simulink model "gtm_aeromodel"  (Simulink 7.2)
settings: Solver=ode45  StartTime=0.0  StopTime=10.0  RelTol=1e-3
undefined symbols (not defined in the file or in its folder): A_BLCG, A_BW, A_CW, A_FSCG, A_FSREF_in, A_SW, A_WLCG, A_WLREF, ALPHA0, bclowb, bclowbx_FMACH, bcmowb, bcmowbx_FHP, bcmowby_FMACH, cda, cdax_FLPDEF, cddr, cddrx_FMACH, cdo, cdox_FLPDEF, cdt1, cdt1x_mach, cdt2, cdt2x_mach, cdto, cdtox_mach, cdwb, cdwbx_FALPHA, cdwby_FMACH, clat, clatfr, clatfrx_FHP, clatfry_FMACH, clatx_mach, clawbfr, clawbfrx_FHP, clawbfry_FMACH, cldefr, cldefrx_FHP, cldefry_FMACH, cldtab, cldtabx_FMACH, clqwb, clqwbfr, clqwbfrx_FHP, clqwbfry_FMACH, clqwbx_mach, cltdd, cltddx_FHP, cltddy_FMACH, clwb, clwbtdd, clwbtddx_FHP, clwbtddy_FMACH, clwbx_FALPHA, clwby_FMACH, clwbzdd, clwbzddx_FHP, clwbzddy_FMACH, clzdd ... (+196)
libraries: model_lib x1
(part 3 of 10)

== system gtm_aeromodel/get aero forces and moments/AERODYNAMICS/Aero Incidence Angles/DOWNWASH/epswb_plus_alphadot ==
  mach : Inport  OutDataType=sfix(16)  OutScaling=2^0
  "alpha " : Inport  Port=2  OutDataType=sfix(16)  OutScaling=2^0
  altitude : Inport  Port=3  OutDataType=sfix(16)  OutScaling=2^0
  flex : Inport  Port=4  OutDataType=sfix(16)  OutScaling=2^0
  TAS : Inport  Port=5  OutDataType=sfix(16)  OutScaling=2^0
  alphadot : Inport  Port=6  OutDataType=sfix(16)  OutScaling=2^0
  CMAT : Subsystem  mask(1-D Table){z=CMATx_mach, tab=CMAT}
      mask prompts: z "Z vector:"; tab "Table:"
      mask help: 1-D Table Look Up. Enter monotonic Z vector amd table. See the help for more info.
      mask Help: The Z vector must be monotonic.  Z indexes into the columns of the 1-D tables.   Table does not extrapolate beyound the break vectors
      mask Display: plot(@2)
  Fcn : Fcn  Expr=1/u
  Fcn2 : Fcn  Expr=1/u
  Product{,1..2,4} (4 alike) : Product  OutDataType=sfix(16)  OutScaling=2^0  SaturateOnIntegerOverflow=on  RndMeth=Zero  InputSameDT=on  OutDataTypeStr=Inherit: Same as first input
  Product3 : Product  Inputs=3  OutDataType=sfix(16)  OutScaling=2^0  SaturateOnIntegerOverflow=on  RndMeth=Zero  InputSameDT=on  OutDataTypeStr=Inherit: Same as first input
  Sum1 : Sum  OutDataType=sfix(16)  OutScaling=2^0  SaturateOnIntegerOverflow=on  InputSameDT=on  OutDataTypeStr=Inherit: Same as first input
  Switch6 : Switch  Threshold=0.5  SaturateOnIntegerOverflow=on  InputSameDT=on
  Switch7 : Switch  Threshold=0.5  SaturateOnIntegerOverflow=on  InputSameDT=on
  Switch8 : Switch  Threshold=0.5  SaturateOnIntegerOverflow=on  InputSameDT=on
  clat : Subsystem  mask(1-D Table){z=clatx_mach, tab=clat}
      mask prompts: z "Z vector:"; tab "Table:"
      mask help: 1-D Table Look Up. Enter monotonic Z vector amd table. See the help for more info.
      mask Help: The Z vector must be monotonic.  Z indexes into the columns of the 1-D tables.   Table does not extrapolate beyound the break vectors
      mask Display: plot(@2)
  despoflex : Subsystem  TreatAsAtomicUnit=on
  epsa : Subsystem  mask(1-D Table){z=epsax_mach, tab=epsa}
      mask prompts: z "Z vector:"; tab "Table:"
      mask help: 1-D Table Look Up. Enter monotonic Z vector amd table. See the help for more info.
      mask Help: The Z vector must be monotonic.  Z indexes into the columns of the 1-D tables.   Table does not extrapolate beyound the break vectors
      mask Display: plot(@2)
  epsad : Gain  Gain=-1  ParameterDataType=sfix(16)  ParameterScaling=2^0  OutDataType=sfix(16)  OutScaling=2^0  SaturateOnIntegerOverflow=on  OutDataTypeStr=Inherit: Same as input  ParamDataTypeStr=Inherit: Same as input
  epso : Sum  OutDataType=sfix(16)  OutScaling=2^0  SaturateOnIntegerOverflow=on  InputSameDT=on  OutDataTypeStr=Inherit: Same as first input
  epsodsb : Subsystem  mask(2-D Table){y=epsodsbx_DSB, z=epsodsby_FMACH, tab=epsodsb}
      mask prompts: y "Y vector:"; z "Z vector:"; tab "Table:"
      mask help: 2-D Table Look Up. Enter monotonic Y and Z vectors and a matrix of 2-D tables. See the help for more info.
      mask Help: The Y and Z vectors must be monotonic.  Y  indexes into the columns of the 2-D table & Z indexes into the rows of the 2-D tables.   The input values are y and z respectively (e.g., top port = y).
      mask Display: plot(-10,-10,110,110,[90,50,10],[90,40,30],[90,50,10],[50,26,20],[90,50,10],[22,13,10])
  one : Constant  Value=1.0  OutDataType=sfix(16)  OutScaling=2^0
  one1 : Constant  Value=A_CW  OutDataType=sfix(16)  OutScaling=2^0
  r2d : Gain  Gain=constants.r2d  ParameterDataType=sfix(16)  ParameterScaling=2^0  OutDataType=sfix(16)  OutScaling=2^0  SaturateOnIntegerOverflow=on  OutDataTypeStr=Inherit: Same as input  ParamDataTypeStr=Inherit: Same as input
  xht_ : Gain  Gain=-1  ParameterDataType=sfix(16)  ParameterScaling=2^0  OutDataType=sfix(16)  OutScaling=2^0  SaturateOnIntegerOverflow=on  OutDataTypeStr=Inherit: Same as input  ParamDataTypeStr=Inherit: Same as input
  xhtp : Product  Inputs=3  OutDataType=sfix(16)  OutScaling=2^0  SaturateOnIntegerOverflow=on  RndMeth=Zero  InputSameDT=on  OutDataTypeStr=Inherit: Same as first input
  zero : Constant  Value=0.0  OutDataType=sfix(16)  OutScaling=2^0
  zero1 : Constant  Value=0.0  OutDataType=sfix(16)  OutScaling=2^0
  epswb : Outport  OutDataType=sfix(16)  OutScaling=2^0  InitialOutput=0
  deps_alpha_dot : Outport  Port=2  OutDataType=sfix(16)  OutScaling=2^0  InitialOutput=0
  xht : Outport  Port=3  OutDataType=sfix(16)  OutScaling=2^0  InitialOutput=0
  wires:
  epsad/1 -> deps_alpha_dot/1
  Product4/1 -> epsad/1
  r2d/1 -> Product3/3
  alphadot/1 -> r2d/1
  epsodsb/1(Interp Value) -> epso/2
  Switch6/1 -> epso/1
  Switch7/1 -> Product/2
  epsa/1(Interp Value) -> Product/1
  TAS/1 -> Fcn2/1
  Product1/1 -> Product4/1, Sum1/1
  Fcn2/1 -> Product3/2
  Product2/1 -> xhtp/2
  Switch8/1 -> xhtp/1
  Fcn/1 -> Product2/2
  CMAT/1(Interp Value) -> Product2/1
  clat/1(Interp Value) -> Fcn/1
  one/1 -> Switch8/3, Switch7/3
  despoflex/2(cmocl_atr) -> Switch8/1
  despoflex/1(epsafr) -> Switch7/1
  zero/1 -> epsodsb/1(Y)
  epso/1 -> Sum1/2
  altitude/1 -> despoflex/1(altitude)
  flex/1 -> Switch7/2, Switch8/2, Switch6/2, despoflex/Enable
  zero1/1 -> Switch6/3
  despoflex/3(despoflex) -> Switch6/1
  mach/1 -> epsa/1(Z), clat/1(Z), CMAT/1(Z), epsodsb/2(Z), despoflex/2(Mach)
  Product/1 -> Product1/1
  Sum1/1 -> epswb/1
  xhtp/1 -> xht_/1
  one1/1 -> xhtp/3
  xht_/1 -> Product3/1, xht/1
  Product3/1 -> Product4/2
  "alpha "/1 -> Product1/2

== system gtm_aeromodel/get aero forces and moments/AERODYNAMICS/Aero Incidence Angles/DOWNWASH/sb_df_int ==
  dsb : Inport  OutDataType=sfix(16)  OutScaling=2^0
  alpha : Inport  Port=2  OutDataType=sfix(16)  OutScaling=2^0
  flap : Inport  Port=3  OutDataType=sfix(16)  OutScaling=2^0
  Enable : EnablePort
  Sum1 : Sum  Inputs=-+-+  OutDataType=sfix(16)  OutScaling=2^0  SaturateOnIntegerOverflow=on  InputSameDT=on  OutDataTypeStr=Inherit: Same as first input
  epsdsbdf_ : Subsystem  mask(1-2-3 Table){@1=epsdsbdfx_DSB, @2=epsdsbdfy_FALPHA, @3=epsdsbdfz_FLPDEF, @4=epsdsbdf}
      mask prompts: @1 "X vector:"; @2 "Y vector:"; @3 "Z vector:"; @4 "Table:"
      mask help: 3-D Table Look Up. Enter monotonic X, Y and Z vectors and a matrix of 2-D tables. See the help for more info.
      mask init:
      | x=@1;y=@2;z=@3;tab=@4;
      mask Help: The X, Y and Z vectors must be monotonic.   The 3-D table is a horizontal concatenation of  2-D tables.  X  indexes into the columns of the 2-D tables & Y indexes into the rows of the 2-D tables.  Z indexes into the table levels (starting with the 1st 2-D table).   The input values are x, y and z respectively (e.g., top port = x).
      mask Display: plot([0 2 2 0 0],[0 0 2 2 0],[0 2 2.9 0.95 0],[2 2 2.7 2.7 2],[2 2.9 2.9 2 2],[0 0.85 2.7 2 0])
  epsdsbdf_1 : Subsystem  mask(1-2-3 Table){@1=epsdsbdfx_DSB, @2=epsdsbdfy_FALPHA, @3=epsdsbdfz_FLPDEF, @4=epsdsbdf}
      mask prompts: @1 "X vector:"; @2 "Y vector:"; @3 "Z vector:"; @4 "Table:"
      mask help: 3-D Table Look Up. Enter monotonic X, Y and Z vectors and a matrix of 2-D tables. See the help for more info.
      mask init:
      | x=@1;y=@2;z=@3;tab=@4;
      mask Help: The X, Y and Z vectors must be monotonic.   The 3-D table is a horizontal concatenation of  2-D tables.  X  indexes into the columns of the 2-D tables & Y indexes into the rows of the 2-D tables.  Z indexes into the table levels (starting with the 1st 2-D table).   The input values are x, y and z respectively (e.g., top port = x).
      mask Display: plot([0 2 2 0 0],[0 0 2 2 0],[0 2 2.9 0.95 0],[2 2 2.7 2.7 2],[2 2.9 2.9 2 2],[0 0.85 2.7 2 0])
  epsodsb : Subsystem  mask(2-D Table){y=epsodsbx_DSB, z=epsodsby_FMACH, tab=epsodsb}
      mask prompts: y "Y vector:"; z "Z vector:"; tab "Table:"
      mask help: 2-D Table Look Up. Enter monotonic Y and Z vectors and a matrix of 2-D tables. See the help for more info.
      mask Help: The Y and Z vectors must be monotonic.  Y  indexes into the columns of the 2-D table & Z indexes into the rows of the 2-D tables.   The input values are y and z respectively (e.g., top port = y).
      mask Display: plot(-10,-10,110,110,[90,50,10],[90,40,30],[90,50,10],[50,26,20],[90,50,10],[22,13,10])
  epsodsb1 : Subsystem  mask(2-D Table){y=epsodsbx_DSB, z=epsodsby_FMACH, tab=epsodsb}
      mask prompts: y "Y vector:"; z "Z vector:"; tab "Table:"
      mask help: 2-D Table Look Up. Enter monotonic Y and Z vectors and a matrix of 2-D tables. See the help for more info.
      mask Help: The Y and Z vectors must be monotonic.  Y  indexes into the columns of the 2-D table & Z indexes into the rows of the 2-D tables.   The input values are y and z respectively (e.g., top port = y).
      mask Display: plot(-10,-10,110,110,[90,50,10],[90,40,30],[90,50,10],[50,26,20],[90,50,10],[22,13,10])
  mach0 : Constant  Value=.178  OutDataType=sfix(16)  OutScaling=2^0
  mach1 : Constant  Value=0  OutDataType=sfix(16)  OutScaling=2^0
  sb_int_df : Outport  OutDataType=sfix(16)  OutScaling=2^0  InitialOutput=0
  wires:
  Sum1/1 -> sb_int_df/1
  dsb/1 -> epsodsb/1(Y), epsdsbdf_/1(X)
  epsodsb1/1(Interp Value) -> Sum1/4
  epsodsb/1(Interp Value) -> Sum1/3
  epsdsbdf_/1(Interp Value) -> Sum1/2
  epsdsbdf_1/1(Interp Value) -> Sum1/1
  alpha/1 -> epsdsbdf_/2(Y), epsdsbdf_1/2(Y)
  flap/1 -> epsdsbdf_/3(Z), epsdsbdf_1/3(Z)
  mach1/1 -> epsdsbdf_1/1(X), epsodsb1/1(Y)
  mach0/1 -> epsodsb/2(Z), epsodsb1/2(Z)

== system gtm_aeromodel/get aero forces and moments/AERODYNAMICS/Aero Incidence Angles/DOWNWASH/sp_int ==
  dsl : Inport  OutDataType=sfix(16)  OutScaling=2^0
  alpha : Inport  Port=2  OutDataType=sfix(16)  OutScaling=2^0
  flap : Inport  Port=3  OutDataType=sfix(16)  OutScaling=2^0
  dsb : Inport  Port=4  OutDataType=sfix(16)  OutScaling=2^0
  dsr : Inport  Port=5  OutDataType=sfix(16)  OutScaling=2^0
  Enable : EnablePort
  Constant17 : Constant  Value=2  OutDataType=sfix(16)  OutScaling=2^0
  Sum4 : Sum  Inputs=++--+-  OutDataType=sfix(16)  OutScaling=2^0  SaturateOnIntegerOverflow=on  InputSameDT=on  OutDataTypeStr=Inherit: Same as first input
  eps_spoiler : Product  OutDataType=sfix(16)  OutScaling=2^0  SaturateOnIntegerOverflow=on  RndMeth=Zero  InputSameDT=on  OutDataTypeStr=Inherit: Same as first input
  eps_spoiler1 : Product  OutDataType=sfix(16)  OutScaling=2^0  SaturateOnIntegerOverflow=on  RndMeth=Zero  InputSameDT=on  OutDataTypeStr=Inherit: Same as first input
  epsdsldf : Subsystem  mask(1-2-3 Table){@1=epsdsldfx_DSL, @2=epsdsldfy_FALPHA, @3=epsdsldfz_FLPDEF, @4=epsdsldf}
      mask prompts: @1 "X vector:"; @2 "Y vector:"; @3 "Z vector:"; @4 "Table:"
      mask help: 3-D Table Look Up. Enter monotonic X, Y and Z vectors and a matrix of 2-D tables. See the help for more info.
      mask init:
      | x=@1;y=@2;z=@3;tab=@4;
      mask Help: The X, Y and Z vectors must be monotonic.   The 3-D table is a horizontal concatenation of  2-D tables.  X  indexes into the columns of the 2-D tables & Y indexes into the rows of the 2-D tables.  Z indexes into the table levels (starting with the 1st 2-D table).   The input values are x, y and z respectively (e.g., top port = x).
      mask Display: plot([0 2 2 0 0],[0 0 2 2 0],[0 2 2.9 0.95 0],[2 2 2.7 2.7 2],[2 2.9 2.9 2 2],[0 0.85 2.7 2 0])
  epsdsldf1 : Subsystem  mask(1-2-3 Table){@1=epsdsldfx_DSL, @2=epsdsldfy_FALPHA, @3=epsdsldfz_FLPDEF, @4=epsdsldf}
      mask prompts: @1 "X vector:"; @2 "Y vector:"; @3 "Z vector:"; @4 "Table:"
      mask help: 3-D Table Look Up. Enter monotonic X, Y and Z vectors and a matrix of 2-D tables. See the help for more info.
      mask init:
      | x=@1;y=@2;z=@3;tab=@4;
      mask Help: The X, Y and Z vectors must be monotonic.   The 3-D table is a horizontal concatenation of  2-D tables.  X  indexes into the columns of the 2-D tables & Y indexes into the rows of the 2-D tables.  Z indexes into the table levels (starting with the 1st 2-D table).   The input values are x, y and z respectively (e.g., top port = x).
      mask Display: plot([0 2 2 0 0],[0 0 2 2 0],[0 2 2.9 0.95 0],[2 2 2.7 2.7 2],[2 2.9 2.9 2 2],[0 0.85 2.7 2 0])
  epsdsldf2 : Subsystem  mask(1-2-3 Table){@1=epsdsldfx_DSL, @2=epsdsldfy_FALPHA, @3=epsdsldfz_FLPDEF, @4=epsdsldf}
      mask prompts: @1 "X vector:"; @2 "Y vector:"; @3 "Z vector:"; @4 "Table:"
      mask help: 3-D Table Look Up. Enter monotonic X, Y and Z vectors and a matrix of 2-D tables. See the help for more info.
      mask init:
      | x=@1;y=@2;z=@3;tab=@4;
      mask Help: The X, Y and Z vectors must be monotonic.   The 3-D table is a horizontal concatenation of  2-D tables.  X  indexes into the columns of the 2-D tables & Y indexes into the rows of the 2-D tables.  Z indexes into the table levels (starting with the 1st 2-D table).   The input values are x, y and z respectively (e.g., top port = x).
      mask Display: plot([0 2 2 0 0],[0 0 2 2 0],[0 2 2.9 0.95 0],[2 2 2.7 2.7 2],[2 2.9 2.9 2 2],[0 0.85 2.7 2 0])
  epsodsl : Subsystem  mask(2-D Table){y=epsodslx_DSL, z=epsodsly_FMACH, tab=epsodsl}
      mask prompts: y "Y vector:"; z "Z vector:"; tab "Table:"
      mask help: 2-D Table Look Up. Enter monotonic Y and Z vectors and a matrix of 2-D tables. See the help for more info.
      mask Help: The Y and Z vectors must be monotonic.  Y  indexes into the columns of the 2-D table & Z indexes into the rows of the 2-D tables.   The input values are y and z respectively (e.g., top port = y).
      mask Display: plot(-10,-10,110,110,[90,50,10],[90,40,30],[90,50,10],[50,26,20],[90,50,10],[22,13,10])
  epsodsl1 : Subsystem  mask(2-D Table){y=epsodslx_DSL, z=epsodsly_FMACH, tab=epsodsl}
      mask prompts: y "Y vector:"; z "Z vector:"; tab "Table:"
      mask help: 2-D Table Look Up. Enter monotonic Y and Z vectors and a matrix of 2-D tables. See the help for more info.
      mask Help: The Y and Z vectors must be monotonic.  Y  indexes into the columns of the 2-D table & Z indexes into the rows of the 2-D tables.   The input values are y and z respectively (e.g., top port = y).
      mask Display: plot(-10,-10,110,110,[90,50,10],[90,40,30],[90,50,10],[50,26,20],[90,50,10],[22,13,10])
  epsodsl2 : Subsystem  mask(2-D Table){y=epsodslx_DSL, z=epsodsly_FMACH, tab=epsodsl}
      mask prompts: y "Y vector:"; z "Z vector:"; tab "Table:"
      mask help: 2-D Table Look Up. Enter monotonic Y and Z vectors and a matrix of 2-D tables. See the help for more info.
      mask Help: The Y and Z vectors must be monotonic.  Y  indexes into the columns of the 2-D table & Z indexes into the rows of the 2-D tables.   The input values are y and z respectively (e.g., top port = y).
      mask Display: plot(-10,-10,110,110,[90,50,10],[90,40,30],[90,50,10],[50,26,20],[90,50,10],[22,13,10])
  mach0 : Constant  Value=0.178  OutDataType=sfix(16)  OutScaling=2^0
  sp_int : Outport  OutDataType=sfix(16)  OutScaling=2^0  InitialOutput=0
  wires:
  flap/1 -> epsdsldf/3(Z), epsdsldf2/3(Z), epsdsldf1/3(Z)
  alpha/1 -> epsdsldf/2(Y), epsdsldf1/2(Y), epsdsldf2/2(Y)
  epsdsldf/1(Interp Value) -> Sum4/2
  epsdsldf2/1(Interp Value) -> Sum4/1
  eps_spoiler/1 -> Sum4/3
  epsdsldf1/1(Interp Value) -> eps_spoiler/2
  dsl/1 -> epsdsldf/1(X), epsodsl/1(Y)
  dsb/1 -> epsdsldf1/1(X), epsodsl2/1(Y)
  mach0/1 -> epsodsl/2(Z), epsodsl2/2(Z), epsodsl1/2(Z)
  dsr/1 -> epsdsldf2/1(X), epsodsl1/1(Y)
  epsodsl/1(Interp Value) -> Sum4/4
  Constant17/1 -> eps_spoiler/1, eps_spoiler1/1
  epsodsl2/1(Interp Value) -> eps_spoiler1/2
  eps_spoiler1/1 -> Sum4/5
  epsodsl1/1(Interp Value) -> Sum4/6
  Sum4/1 -> sp_int/1

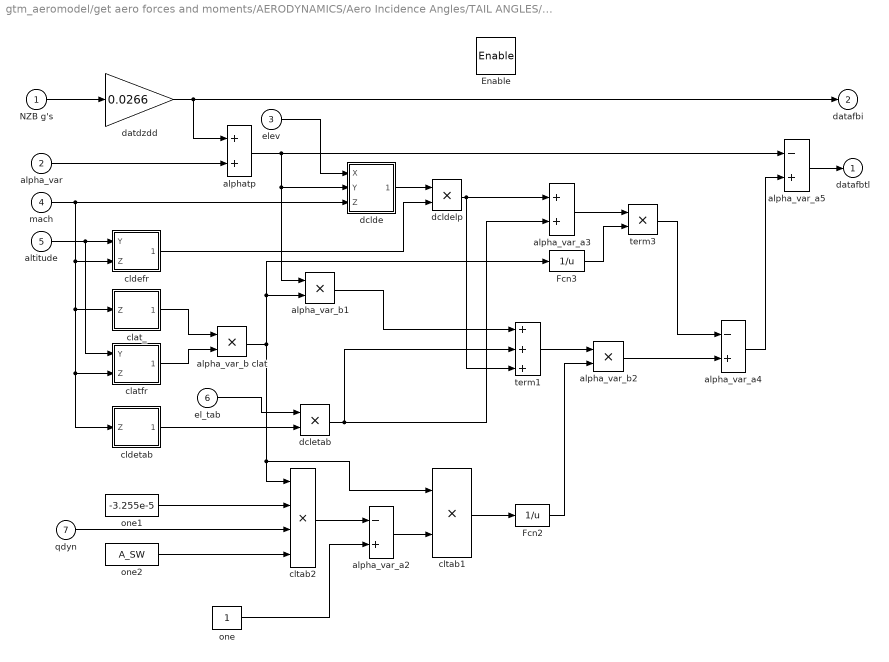
== system gtm_aeromodel/get aero forces and moments/AERODYNAMICS/Aero Incidence Angles/TAIL ANGLES/dalphat_flex ==
  NZB g's : Inport  OutDataType=sfix(16)  OutScaling=2^0
  alpha_var : Inport  Port=2  OutDataType=sfix(16)  OutScaling=2^0
  elev : Inport  Port=3  OutDataType=sfix(16)  OutScaling=2^0
  mach : Inport  Port=4  OutDataType=sfix(16)  OutScaling=2^0
  altitude : Inport  Port=5  OutDataType=sfix(16)  OutScaling=2^0
  el_tab : Inport  Port=6  OutDataType=sfix(16)  OutScaling=2^0
  qdyn : Inport  Port=7  OutDataType=sfix(16)  OutScaling=2^0
  Enable : EnablePort
  Fcn2 : Fcn  Expr=1/u
  Fcn3 : Fcn  Expr=1/u
  alpha_var_a2 : Sum  Inputs=-+  OutDataType=sfix(16)  OutScaling=2^0  SaturateOnIntegerOverflow=on  InputSameDT=on  OutDataTypeStr=Inherit: Same as first input
  alpha_var_a3 : Sum  OutDataType=sfix(16)  OutScaling=2^0  SaturateOnIntegerOverflow=on  InputSameDT=on  OutDataTypeStr=Inherit: Same as first input
  alpha_var_a4 : Sum  Inputs=-+  OutDataType=sfix(16)  OutScaling=2^0  SaturateOnIntegerOverflow=on  InputSameDT=on  OutDataTypeStr=Inherit: Same as first input
  alpha_var_a5 : Sum  Inputs=-+  OutDataType=sfix(16)  OutScaling=2^0  SaturateOnIntegerOverflow=on  InputSameDT=on  OutDataTypeStr=Inherit: Same as first input
  alpha_var_b clat : Product  OutDataType=sfix(16)  OutScaling=2^0  SaturateOnIntegerOverflow=on  RndMeth=Zero  InputSameDT=on  OutDataTypeStr=Inherit: Same as first input
  alpha_var_b1 : Product  OutDataType=sfix(16)  OutScaling=2^0  SaturateOnIntegerOverflow=on  RndMeth=Zero  InputSameDT=on  OutDataTypeStr=Inherit: Same as first input
  alpha_var_b2 : Product  OutDataType=sfix(16)  OutScaling=2^0  SaturateOnIntegerOverflow=on  RndMeth=Zero  InputSameDT=on  OutDataTypeStr=Inherit: Same as first input
  alphatp : Sum  OutDataType=sfix(16)  OutScaling=2^0  SaturateOnIntegerOverflow=on  InputSameDT=on  OutDataTypeStr=Inherit: Same as first input
  clat_ : Subsystem  mask(1-D Table){z=clatx_mach, tab=clat}
      mask prompts: z "Z vector:"; tab "Table:"
      mask help: 1-D Table Look Up. Enter monotonic Z vector amd table. See the help for more info.
      mask Help: The Z vector must be monotonic.  Z indexes into the columns of the 1-D tables.   Table does not extrapolate beyound the break vectors
      mask Display: plot(@2)
  clatfr : Subsystem  mask(2-D Table){y=clatfrx_FHP, z=clatfry_FMACH, tab=clatfr}
      mask prompts: y "Y vector:"; z "Z vector:"; tab "Table:"
      mask help: 2-D Table Look Up. Enter monotonic Y and Z vectors and a matrix of 2-D tables. See the help for more info.
      mask Help: The Y and Z vectors must be monotonic.  Y  indexes into the columns of the 2-D table & Z indexes into the rows of the 2-D tables.   The input values are y and z respectively (e.g., top port = y).
      mask Display: plot(-10,-10,110,110,[90,50,10],[90,40,30],[90,50,10],[50,26,20],[90,50,10],[22,13,10])
  cldefr : Subsystem  mask(2-D Table){y=cldefrx_FHP, z=cldefry_FMACH, tab=cldefr}
      mask prompts: y "Y vector:"; z "Z vector:"; tab "Table:"
      mask help: 2-D Table Look Up. Enter monotonic Y and Z vectors and a matrix of 2-D tables. See the help for more info.
      mask Help: The Y and Z vectors must be monotonic.  Y  indexes into the columns of the 2-D table & Z indexes into the rows of the 2-D tables.   The input values are y and z respectively (e.g., top port = y).
      mask Display: plot(-10,-10,110,110,[90,50,10],[90,40,30],[90,50,10],[50,26,20],[90,50,10],[22,13,10])
  cldetab : Subsystem  mask(1-D Table){z=cldtabx_FMACH, tab=cldtab}
      mask prompts: z "Z vector:"; tab "Table:"
      mask help: 1-D Table Look Up. Enter monotonic Z vector amd table. See the help for more info.
      mask Help: The Z vector must be monotonic.  Z indexes into the columns of the 1-D tables.   Table does not extrapolate beyound the break vectors
      mask Display: plot(@2)
  cltab1 : Product  OutDataType=sfix(16)  OutScaling=2^0  SaturateOnIntegerOverflow=on  RndMeth=Zero  InputSameDT=on  OutDataTypeStr=Inherit: Same as first input
  cltab2 : Product  Inputs=4  OutDataType=sfix(16)  OutScaling=2^0  SaturateOnIntegerOverflow=on  RndMeth=Zero  InputSameDT=on  OutDataTypeStr=Inherit: Same as first input
  datdzdd : Gain  Gain=0.0266  ParameterDataType=sfix(16)  ParameterScaling=2^0  OutDataType=sfix(16)  OutScaling=2^0  SaturateOnIntegerOverflow=on  OutDataTypeStr=Inherit: Same as input  ParamDataTypeStr=Inherit: Same as input
  dclde : Subsystem  mask(1-2-3 Table){@1=dcldex_FELE, @2=dcldey_ALPHAT, @3=dcldez_FMACH, @4=dclde}
      mask prompts: @1 "X vector:"; @2 "Y vector:"; @3 "Z vector:"; @4 "Table:"
      mask help: 3-D Table Look Up. Enter monotonic X, Y and Z vectors and a matrix of 2-D tables. See the help for more info.
      mask init:
      | x=@1;y=@2;z=@3;tab=@4;
      mask Help: The X, Y and Z vectors must be monotonic.   The 3-D table is a horizontal concatenation of  2-D tables.  X  indexes into the columns of the 2-D tables & Y indexes into the rows of the 2-D tables.  Z indexes into the table levels (starting with the 1st 2-D table).   The input values are x, y and z respectively (e.g., top port = x).
      mask Display: plot([0 2 2 0 0],[0 0 2 2 0],[0 2 2.9 0.95 0],[2 2 2.7 2.7 2],[2 2.9 2.9 2 2],[0 0.85 2.7 2 0])
  dcldelp : Product  OutDataType=sfix(16)  OutScaling=2^0  SaturateOnIntegerOverflow=on  RndMeth=Zero  InputSameDT=on  OutDataTypeStr=Inherit: Same as first input
  dcletab : Product  OutDataType=sfix(16)  OutScaling=2^0  SaturateOnIntegerOverflow=on  RndMeth=Zero  InputSameDT=on  OutDataTypeStr=Inherit: Same as first input
  one : Constant  OutDataType=sfix(16)  OutScaling=2^0
  one1 : Constant  Value=-3.255e-5  OutDataType=sfix(16)  OutScaling=2^0
  one2 : Constant  Value=A_SW  OutDataType=sfix(16)  OutScaling=2^0
  term1 : Sum  Inputs=+++  OutDataType=sfix(16)  OutScaling=2^0  SaturateOnIntegerOverflow=on  InputSameDT=on  OutDataTypeStr=Inherit: Same as first input
  term3 : Product  OutDataType=sfix(16)  OutScaling=2^0  SaturateOnIntegerOverflow=on  RndMeth=Zero  InputSameDT=on  OutDataTypeStr=Inherit: Same as first input
  datafbtl : Outport  OutDataType=sfix(16)  OutScaling=2^0  InitialOutput=0
  datafbi : Outport  Port=2  OutDataType=sfix(16)  OutScaling=2^0  InitialOutput=0
  wires:
  cltab1/1 -> Fcn2/1
  cldetab/1(Interp Value) -> dcletab/2
  term1/1 -> alpha_var_b2/1
  term3/1 -> alpha_var_a4/1
  dclde/1(Interp Value) -> dcldelp/1
  NZB g's/1 -> datdzdd/1
  datdzdd/1 -> datafbi/1, alphatp/1
  alpha_var/1 -> alphatp/2
  elev/1 -> dclde/1(X)
  mach/1 -> dclde/3(Z), clat_/1(Z), clatfr/2(Z), cldetab/1(Z), cldefr/2(Z)
  clat_/1(Interp Value) -> alpha_var_b clat/1
  clatfr/1(Interp Value) -> alpha_var_b clat/2
  altitude/1 -> cldefr/1(Y), clatfr/1(Y)
  cldefr/1(Interp Value) -> dcldelp/2
  el_tab/1 -> dcletab/1
  alpha_var_b1/1 -> term1/1
  alpha_var_b clat/1 -> alpha_var_b1/2, Fcn3/1, cltab1/1, cltab2/1
  one/1 -> alpha_var_a2/2
  alpha_var_a2/1 -> cltab1/2
  Fcn2/1 -> alpha_var_b2/2
  dcletab/1 -> term1/2, alpha_var_a3/2
  alpha_var_a3/1 -> term3/1
  Fcn3/1 -> term3/2
  alpha_var_b2/1 -> alpha_var_a4/2
  alphatp/1 -> alpha_var_a5/1, dclde/2(Y), alpha_var_b1/1
  alpha_var_a4/1 -> alpha_var_a5/2
  alpha_var_a5/1 -> datafbtl/1
  dcldelp/1 -> alpha_var_a3/1, term1/3
  cltab2/1 -> alpha_var_a2/1
  one1/1 -> cltab2/2
  qdyn/1 -> cltab2/3
  one2/1 -> cltab2/4

== system gtm_aeromodel/get aero forces and moments/AERODYNAMICS/Aero Incidence Angles/TAIL ANGLES/dbetat_flex ==
  "side acc " : Inport  OutDataType=sfix(16)  OutScaling=2^0
  beta : Inport  Port=2  OutDataType=sfix(16)  OutScaling=2^0
  rud : Inport  Port=3  OutDataType=sfix(16)  OutScaling=2^0
  mach : Inport  Port=4  OutDataType=sfix(16)  OutScaling=2^0
  altitude : Inport  Port=5  OutDataType=sfix(16)  OutScaling=2^0
  qdyn : Inport  Port=6  OutDataType=sfix(16)  OutScaling=2^0
  alpha : Inport  Port=7  OutDataType=sfix(16)  OutScaling=2^0
  Enable : EnablePort
  Fcn2 : Fcn  Expr=1/u
  Fcn3 : Fcn  Expr=1/u
  Gain : Gain  Gain=-5.95e-6  ParameterDataType=sfix(16)  ParameterScaling=2^0  OutDataType=sfix(16)  OutScaling=2^0  SaturateOnIntegerOverflow=on  OutDataTypeStr=Inherit: Same as input  ParamDataTypeStr=Inherit: Same as input
  alpha_var_a2 : Sum  Inputs=-+  OutDataType=sfix(16)  OutScaling=2^0  SaturateOnIntegerOverflow=on  InputSameDT=on  OutDataTypeStr=Inherit: Same as first input
  alpha_var_a4 : Sum  Inputs=-+  OutDataType=sfix(16)  OutScaling=2^0  SaturateOnIntegerOverflow=on  InputSameDT=on  OutDataTypeStr=Inherit: Same as first input
  alpha_var_a5 : Sum  Inputs=-+  OutDataType=sfix(16)  OutScaling=2^0  SaturateOnIntegerOverflow=on  InputSameDT=on  OutDataTypeStr=Inherit: Same as first input
  alpha_var_b1 : Product  Inputs=3  OutDataType=sfix(16)  OutScaling=2^0  SaturateOnIntegerOverflow=on  RndMeth=Zero  InputSameDT=on  OutDataTypeStr=Inherit: Same as first input
  alpha_var_b2 : Product  OutDataType=sfix(16)  OutScaling=2^0  SaturateOnIntegerOverflow=on  RndMeth=Zero  InputSameDT=on  OutDataTypeStr=Inherit: Same as first input
  alpha_var_b3 : Product  OutDataType=sfix(16)  OutScaling=2^0  SaturateOnIntegerOverflow=on  RndMeth=Zero  InputSameDT=on  OutDataTypeStr=Inherit: Same as first input
  beta_var_a : Product  OutDataType=sfix(16)  OutScaling=2^0  SaturateOnIntegerOverflow=on  RndMeth=Zero  InputSameDT=on  OutDataTypeStr=Inherit: Same as first input
  beta_var_b : Product  Inputs=3  OutDataType=sfix(16)  OutScaling=2^0  SaturateOnIntegerOverflow=on  RndMeth=Zero  InputSameDT=on  OutDataTypeStr=Inherit: Same as first input
  cltab1 : Product  Inputs=5  OutDataType=sfix(16)  OutScaling=2^0  SaturateOnIntegerOverflow=on  RndMeth=Zero  InputSameDT=on  OutDataTypeStr=Inherit: Same as first input
  cybfr : Subsystem  mask(2-D Table){y=cybfrx_FHP, z=cybfry_FMACH, tab=cybfr}
      mask prompts: y "Y vector:"; z "Z vector:"; tab "Table:"
      mask help: 2-D Table Look Up. Enter monotonic Y and Z vectors and a matrix of 2-D tables. See the help for more info.
      mask Help: The Y and Z vectors must be monotonic.  Y  indexes into the columns of the 2-D table & Z indexes into the rows of the 2-D tables.   The input values are y and z respectively (e.g., top port = y).
      mask Display: plot(-10,-10,110,110,[90,50,10],[90,40,30],[90,50,10],[50,26,20],[90,50,10],[22,13,10])
  cybvt : Subsystem  mask(2-D Table){y=cybvtx_FMACH, z=cybvty_FALPHA, tab=cybvt}
      mask prompts: y "Y vector:"; z "Z vector:"; tab "Table:"
      mask help: 2-D Table Look Up. Enter monotonic Y and Z vectors and a matrix of 2-D tables. See the help for more info.
      mask Help: The Y and Z vectors must be monotonic.  Y  indexes into the columns of the 2-D table & Z indexes into the rows of the 2-D tables.   The input values are y and z respectively (e.g., top port = y).
      mask Display: plot(-10,-10,110,110,[90,50,10],[90,40,30],[90,50,10],[50,26,20],[90,50,10],[22,13,10])
  cydr : Subsystem  mask(1-D Table){z=cydrx_FMACH, tab=cddr}
      mask prompts: z "Z vector:"; tab "Table:"
      mask help: 1-D Table Look Up. Enter monotonic Z vector amd table. See the help for more info.
      mask Help: The Z vector must be monotonic.  Z indexes into the columns of the 1-D tables.   Table does not extrapolate beyound the break vectors
      mask Display: plot(@2)
  cydrfr : Subsystem  mask(2-D Table){y=cydrfrx_FHP, z=cydrfry_FMACH, tab=cydrfr}
      mask prompts: y "Y vector:"; z "Z vector:"; tab "Table:"
      mask help: 2-D Table Look Up. Enter monotonic Y and Z vectors and a matrix of 2-D tables. See the help for more info.
      mask Help: The Y and Z vectors must be monotonic.  Y  indexes into the columns of the 2-D table & Z indexes into the rows of the 2-D tables.   The input values are y and z respectively (e.g., top port = y).
      mask Display: plot(-10,-10,110,110,[90,50,10],[90,40,30],[90,50,10],[50,26,20],[90,50,10],[22,13,10])
  one : Constant  OutDataType=sfix(16)  OutScaling=2^0
  one1 : Constant  Value=1.07e-5  OutDataType=sfix(16)  OutScaling=2^0
  one2 : Constant  Value=A_SW  OutDataType=sfix(16)  OutScaling=2^0
  dbetat_tail_bend : Outport  OutDataType=sfix(16)  OutScaling=2^0  InitialOutput=0
  dbetat_fus_bend : Outport  Port=2  OutDataType=sfix(16)  OutScaling=2^0  InitialOutput=0
  wires:
  alpha_var_b3/1 -> alpha_var_a4/1
  Fcn3/1 -> alpha_var_b3/2
  beta_var_b/1 -> alpha_var_b3/1, alpha_var_b1/2
  mach/1 -> cydr/1(Z), cybfr/1(Y), cybvt/1(Y), cybfr/2(Z), cydrfr/2(Z)
  beta/1 -> alpha_var_b1/1, alpha_var_a5/1
  Gain/1 -> dbetat_fus_bend/1
  cydr/1(Interp Value) -> beta_var_b/1
  cydrfr/1(Interp Value) -> beta_var_b/3
  rud/1 -> beta_var_b/2
  altitude/1 -> cydrfr/1(Y)
  alpha/1 -> cybvt/2(Z)
  cybvt/1(Interp Value) -> beta_var_a/2
  cybfr/1(Interp Value) -> beta_var_a/1
  alpha_var_b1/1 -> alpha_var_b2/1
  alpha_var_a5/1 -> dbetat_tail_bend/1
  alpha_var_a4/1 -> alpha_var_a5/2
  alpha_var_b2/1 -> alpha_var_a4/2
  Fcn2/1 -> alpha_var_b2/2
  cltab1/1 -> Fcn2/1
  one2/1 -> cltab1/5
  qdyn/1 -> cltab1/4
  one1/1 -> cltab1/3
  alpha_var_a2/1 -> cltab1/2
  one/1 -> alpha_var_a2/2
  beta_var_a/1 -> Fcn3/1, alpha_var_b1/3, cltab1/1, alpha_var_a2/1
  "side acc "/1 -> Gain/1

== system gtm_aeromodel/get aero forces and moments/AERODYNAMICS/Force  Coefficients/DRAG /CDAIL ==
  aill : Inport  OutDataType=sfix(16)  OutScaling=2^0
  ailr : Inport  Port=2  OutDataType=sfix(16)  OutScaling=2^0
  Sum2 : Sum  OutDataType=sfix(16)  OutScaling=2^0  SaturateOnIntegerOverflow=on  InputSameDT=on  OutDataTypeStr=Inherit: Same as first input
  dcdda : Subsystem  mask(1-D Table){z=dcddax_FAIL, tab=dcdda}
      mask prompts: z "Z vector:"; tab "Table:"
      mask help: 1-D Table Look Up. Enter monotonic Z vector amd table. See the help for more info.
      mask Help: The Z vector must be monotonic.  Z indexes into the columns of the 1-D tables.   Table does not extrapolate beyound the break vectors
      mask Display: plot(@2)
  dcdda1 : Subsystem  mask(1-D Table){z=dcddax_FAIL, tab=dcdda}
      mask prompts: z "Z vector:"; tab "Table:"
      mask help: 1-D Table Look Up. Enter monotonic Z vector amd table. See the help for more info.
      mask Help: The Z vector must be monotonic.  Z indexes into the columns of the 1-D tables.   Table does not extrapolate beyound the break vectors
      mask Display: plot(@2)
  cdail : Outport  OutDataType=sfix(16)  OutScaling=2^0  InitialOutput=0
  wires:
  dcdda1/1(Interp Value) -> Sum2/2
  dcdda/1(Interp Value) -> Sum2/1
  Sum2/1 -> cdail/1
  ailr/1 -> dcdda1/1(Z)
  aill/1 -> dcdda/1(Z)

== system gtm_aeromodel/get aero forces and moments/AERODYNAMICS/Force  Coefficients/DRAG /CDGE ==
  hob : Inport  OutDataType=sfix(16)  OutScaling=2^0
  alpha : Inport  Port=2  OutDataType=sfix(16)  OutScaling=2^0
  flap : Inport  Port=3  OutDataType=sfix(16)  OutScaling=2^0
  dcdhob : Subsystem  mask(1-2-3 Table){@1=dcdhobx_HOB, @2=dcdhoby_FALPHA, @3=dcdhobz_FLPDEF, @4=dcdhob}
      mask prompts: @1 "X vector:"; @2 "Y vector:"; @3 "Z vector:"; @4 "Table:"
      mask help: 3-D Table Look Up. Enter monotonic X, Y and Z vectors and a matrix of 2-D tables. See the help for more info.
      mask init:
      | x=@1;y=@2;z=@3;tab=@4;
      mask Help: The X, Y and Z vectors must be monotonic.   The 3-D table is a horizontal concatenation of  2-D tables.  X  indexes into the columns of the 2-D tables & Y indexes into the rows of the 2-D tables.  Z indexes into the table levels (starting with the 1st 2-D table).   The input values are x, y and z respectively (e.g., top port = x).
      mask Display: plot([0 2 2 0 0],[0 0 2 2 0],[0 2 2.9 0.95 0],[2 2 2.7 2.7 2],[2 2.9 2.9 2 2],[0 0.85 2.7 2 0])
  cdge : Outport  OutDataType=sfix(16)  OutScaling=2^0  InitialOutput=0
  wires:
  hob/1 -> dcdhob/1(X)
  alpha/1 -> dcdhob/2(Y)
  flap/1 -> dcdhob/3(Z)
  dcdhob/1(Interp Value) -> cdge/1

== system gtm_aeromodel/get aero forces and moments/AERODYNAMICS/Force  Coefficients/DRAG /CDGEAR ==
  flap : Inport  OutDataType=sfix(16)  OutScaling=2^0
  alpha : Inport  Port=2  OutDataType=sfix(16)  OutScaling=2^0
  gear : Inport  Port=3  OutDataType=sfix(16)  OutScaling=2^0
  Product : Product  OutDataType=sfix(16)  OutScaling=2^0  SaturateOnIntegerOverflow=on  RndMeth=Zero  InputSameDT=on  OutDataTypeStr=Inherit: Same as first input
  Sum1 : Sum  OutDataType=sfix(16)  OutScaling=2^0  SaturateOnIntegerOverflow=on  InputSameDT=on  OutDataTypeStr=Inherit: Same as first input
  Switch6 : Switch  Threshold=0.5  SaturateOnIntegerOverflow=on  InputSameDT=on
  cda : Subsystem  mask(1-D Table){z=cdax_FLPDEF, tab=cda}
      mask prompts: z "Z vector:"; tab "Table:"
      mask help: 1-D Table Look Up. Enter monotonic Z vector amd table. See the help for more info.
      mask Help: The Z vector must be monotonic.  Z indexes into the columns of the 1-D tables.   Table does not extrapolate beyound the break vectors
      mask Display: plot(@2)
  cdo : Subsystem  mask(1-D Table){z=cdox_FLPDEF, tab=cdo}
      mask prompts: z "Z vector:"; tab "Table:"
      mask help: 1-D Table Look Up. Enter monotonic Z vector amd table. See the help for more info.
      mask Help: The Z vector must be monotonic.  Z indexes into the columns of the 1-D tables.   Table does not extrapolate beyound the break vectors
      mask Display: plot(@2)
  constant1 : Constant  Value=0.0  OutDataType=sfix(16)  OutScaling=2^0
  cdg : Outport  OutDataType=sfix(16)  OutScaling=2^0  InitialOutput=0
  wires:
  flap/1 -> cdo/1(Z), cda/1(Z)
  cda/1(Interp Value) -> Product/1
  alpha/1 -> Product/2
  Product/1 -> Sum1/2
  cdo/1(Interp Value) -> Sum1/1
  Sum1/1 -> Switch6/1
  gear/1 -> Switch6/2
  constant1/1 -> Switch6/3
  Switch6/1 -> cdg/1

== system gtm_aeromodel/get aero forces and moments/AERODYNAMICS/Force  Coefficients/DRAG /CDR ==
  mach : Inport  OutDataType=sfix(16)  OutScaling=2^0
  rud : Inport  Port=2  OutDataType=sfix(16)  OutScaling=2^0
  Fcn : Fcn  Expr=abs(u)
  Product : Product  OutDataType=sfix(16)  OutScaling=2^0  SaturateOnIntegerOverflow=on  RndMeth=Zero  InputSameDT=on  OutDataTypeStr=Inherit: Same as first input
  cddr : Subsystem  mask(1-D Table){z=cddrx_FMACH, tab=cddr}
      mask prompts: z "Z vector:"; tab "Table:"
      mask help: 1-D Table Look Up. Enter monotonic Z vector amd table. See the help for more info.
      mask Help: The Z vector must be monotonic.  Z indexes into the columns of the 1-D tables.   Table does not extrapolate beyound the break vectors
      mask Display: plot(@2)
  cdrud : Outport  OutDataType=sfix(16)  OutScaling=2^0  InitialOutput=0
  wires:
  mach/1 -> cddr/1(Z)
  cddr/1(Interp Value) -> Product/1
  rud/1 -> Fcn/1
  Fcn/1 -> Product/2
  Product/1 -> cdrud/1

== system gtm_aeromodel/get aero forces and moments/AERODYNAMICS/Force  Coefficients/DRAG /CDSPOIL ==
  dsb : Inport  OutDataType=sfix(16)  OutScaling=2^0
  dsl : Inport  Port=2  OutDataType=sfix(16)  OutScaling=2^0
  alpha : Inport  Port=3  OutDataType=sfix(16)  OutScaling=2^0
  mach : Inport  Port=4  OutDataType=sfix(16)  OutScaling=2^0
  flap : Inport  Port=5  OutDataType=sfix(16)  OutScaling=2^0
  dsr : Inport  Port=6  OutDataType=sfix(16)  OutScaling=2^0
  MACH : Constant  Value=.178  OutDataType=sfix(16)  OutScaling=2^0
  Sum1 : Sum  Inputs=-+  OutDataType=sfix(16)  OutScaling=2^0  SaturateOnIntegerOverflow=on  InputSameDT=on  OutDataTypeStr=Inherit: Same as first input
  Sum2 : Sum  OutDataType=sfix(16)  OutScaling=2^0  SaturateOnIntegerOverflow=on  InputSameDT=on  OutDataTypeStr=Inherit: Same as first input
  Sum5 : Sum  Inputs=+-  OutDataType=sfix(16)  OutScaling=2^0  SaturateOnIntegerOverflow=on  InputSameDT=on  OutDataTypeStr=Inherit: Same as first input
  Sum6 : Sum  Inputs=+-  OutDataType=sfix(16)  OutScaling=2^0  SaturateOnIntegerOverflow=on  InputSameDT=on  OutDataTypeStr=Inherit: Same as first input
  Sum7 : Sum  Inputs=+-  OutDataType=sfix(16)  OutScaling=2^0  SaturateOnIntegerOverflow=on  InputSameDT=on  OutDataTypeStr=Inherit: Same as first input
  Switch7 : Switch  Threshold=0.5  SaturateOnIntegerOverflow=on  InputSameDT=on
  Switch8 : Switch  Threshold=0.5  SaturateOnIntegerOverflow=on  InputSameDT=on
  cd_sp_int : Subsystem  TreatAsAtomicUnit=on
  dcdpfint : Sum  Inputs=-+  OutDataType=sfix(16)  OutScaling=2^0  SaturateOnIntegerOverflow=on  InputSameDT=on  OutDataTypeStr=Inherit: Same as first input
  dcdwbdsb : Subsystem  mask(1-2-3 Table){@1=dcdwbdsbx_DSB, @2=dcdwbdsby_ALPHA, @3=dcdwbdsbz_FMACH, @4=dcdwbdsb}
      mask prompts: @1 "X vector:"; @2 "Y vector:"; @3 "Z vector:"; @4 "Table:"
      mask help: 3-D Table Look Up. Enter monotonic X, Y and Z vectors and a matrix of 2-D tables. See the help for more info.
      mask init:
      | x=@1;y=@2;z=@3;tab=@4;
      mask Help: The X, Y and Z vectors must be monotonic.   The 3-D table is a horizontal concatenation of  2-D tables.  X  indexes into the columns of the 2-D tables & Y indexes into the rows of the 2-D tables.  Z indexes into the table levels (starting with the 1st 2-D table).   The input values are x, y and z respectively (e.g., top port = x).
      mask Display: plot([0 2 2 0 0],[0 0 2 2 0],[0 2 2.9 0.95 0],[2 2 2.7 2.7 2],[2 2.9 2.9 2 2],[0 0.85 2.7 2 0])
  dcdwbdsb_ : Subsystem  mask(1-2-3 Table){@1=dcdwbdsbx_DSB, @2=dcdwbdsby_ALPHA, @3=dcdwbdsbz_FMACH, @4=dcdwbdsb}
      mask prompts: @1 "X vector:"; @2 "Y vector:"; @3 "Z vector:"; @4 "Table:"
      mask help: 3-D Table Look Up. Enter monotonic X, Y and Z vectors and a matrix of 2-D tables. See the help for more info.
      mask init:
      | x=@1;y=@2;z=@3;tab=@4;
      mask Help: The X, Y and Z vectors must be monotonic.   The 3-D table is a horizontal concatenation of  2-D tables.  X  indexes into the columns of the 2-D tables & Y indexes into the rows of the 2-D tables.  Z indexes into the table levels (starting with the 1st 2-D table).   The input values are x, y and z respectively (e.g., top port = x).
      mask Display: plot([0 2 2 0 0],[0 0 2 2 0],[0 2 2.9 0.95 0],[2 2 2.7 2.7 2],[2 2.9 2.9 2 2],[0 0.85 2.7 2 0])
  dcdwbdsl : Subsystem  mask(1-2-3 Table){@1=dcdwbdslx_DSL, @2=dcdwbdsly_FALPHA, @3=dcdwbdslz_FMACH, @4=dcdwbdsl}
      mask prompts: @1 "X vector:"; @2 "Y vector:"; @3 "Z vector:"; @4 "Table:"
      mask help: 3-D Table Look Up. Enter monotonic X, Y and Z vectors and a matrix of 2-D tables. See the help for more info.
      mask init:
      | x=@1;y=@2;z=@3;tab=@4;
      mask Help: The X, Y and Z vectors must be monotonic.   The 3-D table is a horizontal concatenation of  2-D tables.  X  indexes into the columns of the 2-D tables & Y indexes into the rows of the 2-D tables.  Z indexes into the table levels (starting with the 1st 2-D table).   The input values are x, y and z respectively (e.g., top port = x).
      mask Display: plot([0 2 2 0 0],[0 0 2 2 0],[0 2 2.9 0.95 0],[2 2 2.7 2.7 2],[2 2.9 2.9 2 2],[0 0.85 2.7 2 0])
  dcdwbdsl1 : Subsystem  mask(1-2-3 Table){@1=dcdwbdslx_DSL, @2=dcdwbdsly_FALPHA, @3=dcdwbdslz_FMACH, @4=dcdwbdsl}
      mask prompts: @1 "X vector:"; @2 "Y vector:"; @3 "Z vector:"; @4 "Table:"
      mask help: 3-D Table Look Up. Enter monotonic X, Y and Z vectors and a matrix of 2-D tables. See the help for more info.
      mask init:
      | x=@1;y=@2;z=@3;tab=@4;
      mask Help: The X, Y and Z vectors must be monotonic.   The 3-D table is a horizontal concatenation of  2-D tables.  X  indexes into the columns of the 2-D tables & Y indexes into the rows of the 2-D tables.  Z indexes into the table levels (starting with the 1st 2-D table).   The input values are x, y and z respectively (e.g., top port = x).
      mask Display: plot([0 2 2 0 0],[0 0 2 2 0],[0 2 2.9 0.95 0],[2 2 2.7 2.7 2],[2 2.9 2.9 2 2],[0 0.85 2.7 2 0])
  dcdwbdsl_ : Subsystem  mask(1-2-3 Table){@1=dcdwbdslx_DSL, @2=dcdwbdsly_FALPHA, @3=dcdwbdslz_FMACH, @4=dcdwbdsl}
      mask prompts: @1 "X vector:"; @2 "Y vector:"; @3 "Z vector:"; @4 "Table:"
      mask help: 3-D Table Look Up. Enter monotonic X, Y and Z vectors and a matrix of 2-D tables. See the help for more info.
      mask init:
      | x=@1;y=@2;z=@3;tab=@4;
      mask Help: The X, Y and Z vectors must be monotonic.   The 3-D table is a horizontal concatenation of  2-D tables.  X  indexes into the columns of the 2-D tables & Y indexes into the rows of the 2-D tables.  Z indexes into the table levels (starting with the 1st 2-D table).   The input values are x, y and z respectively (e.g., top port = x).
      mask Display: plot([0 2 2 0 0],[0 0 2 2 0],[0 2 2.9 0.95 0],[2 2 2.7 2.7 2],[2 2.9 2.9 2 2],[0 0.85 2.7 2 0])
  dcdwbdsl_1 : Subsystem  mask(1-2-3 Table){@1=dcdwbdslx_DSL, @2=dcdwbdsly_FALPHA, @3=dcdwbdslz_FMACH, @4=dcdwbdsl}
      mask prompts: @1 "X vector:"; @2 "Y vector:"; @3 "Z vector:"; @4 "Table:"
      mask help: 3-D Table Look Up. Enter monotonic X, Y and Z vectors and a matrix of 2-D tables. See the help for more info.
      mask init:
      | x=@1;y=@2;z=@3;tab=@4;
      mask Help: The X, Y and Z vectors must be monotonic.   The 3-D table is a horizontal concatenation of  2-D tables.  X  indexes into the columns of the 2-D tables & Y indexes into the rows of the 2-D tables.  Z indexes into the table levels (starting with the 1st 2-D table).   The input values are x, y and z respectively (e.g., top port = x).
      mask Display: plot([0 2 2 0 0],[0 0 2 2 0],[0 2 2.9 0.95 0],[2 2 2.7 2.7 2],[2 2.9 2.9 2 2],[0 0.85 2.7 2 0])
  dcdwbdsl_2 : Subsystem  mask(1-2-3 Table){@1=dcdwbdslx_DSL, @2=dcdwbdsly_FALPHA, @3=dcdwbdslz_FMACH, @4=dcdwbdsl}
      mask prompts: @1 "X vector:"; @2 "Y vector:"; @3 "Z vector:"; @4 "Table:"
      mask help: 3-D Table Look Up. Enter monotonic X, Y and Z vectors and a matrix of 2-D tables. See the help for more info.
      mask init:
      | x=@1;y=@2;z=@3;tab=@4;
      mask Help: The X, Y and Z vectors must be monotonic.   The 3-D table is a horizontal concatenation of  2-D tables.  X  indexes into the columns of the 2-D tables & Y indexes into the rows of the 2-D tables.  Z indexes into the table levels (starting with the 1st 2-D table).   The input values are x, y and z respectively (e.g., top port = x).
      mask Display: plot([0 2 2 0 0],[0 0 2 2 0],[0 2 2.9 0.95 0],[2 2 2.7 2.7 2],[2 2.9 2.9 2 2],[0 0.85 2.7 2 0])
  dcdwbdsl_3 : Subsystem  mask(1-2-3 Table){@1=dcdwbdslx_DSL, @2=dcdwbdsly_FALPHA, @3=dcdwbdslz_FMACH, @4=dcdwbdsl}
      mask prompts: @1 "X vector:"; @2 "Y vector:"; @3 "Z vector:"; @4 "Table:"
      mask help: 3-D Table Look Up. Enter monotonic X, Y and Z vectors and a matrix of 2-D tables. See the help for more info.
      mask init:
      | x=@1;y=@2;z=@3;tab=@4;
      mask Help: The X, Y and Z vectors must be monotonic.   The 3-D table is a horizontal concatenation of  2-D tables.  X  indexes into the columns of the 2-D tables & Y indexes into the rows of the 2-D tables.  Z indexes into the table levels (starting with the 1st 2-D table).   The input values are x, y and z respectively (e.g., top port = x).
      mask Display: plot([0 2 2 0 0],[0 0 2 2 0],[0 2 2.9 0.95 0],[2 2 2.7 2.7 2],[2 2.9 2.9 2 2],[0 0.85 2.7 2 0])
  dclpfint1 : Sum  Inputs=-+  OutDataType=sfix(16)  OutScaling=2^0  SaturateOnIntegerOverflow=on  InputSameDT=on  OutDataTypeStr=Inherit: Same as first input
  dclpfint2 : Sum  Inputs=-+  OutDataType=sfix(16)  OutScaling=2^0  SaturateOnIntegerOverflow=on  InputSameDT=on  OutDataTypeStr=Inherit: Same as first input
  zero : Constant  Value=0.0  OutDataType=sfix(16)  OutScaling=2^0
  cd_spoil : Outport  OutDataType=sfix(16)  OutScaling=2^0  InitialOutput=0
  cd_sb : Outport  Port=2  OutDataType=sfix(16)  OutScaling=2^0  InitialOutput=0
  cd_sp_int_df : Outport  Port=3  OutDataType=sfix(16)  OutScaling=2^0  InitialOutput=0
  wires:
  dcdwbdsb_/1(Interp Value) -> Switch8/1
  dcdwbdsb/1(Interp Value) -> Switch8/3
  dcdwbdsl1/1(Interp Value) -> Sum5/2, Sum1/1
  MACH/1 -> dcdwbdsb_/3(Z), dcdwbdsl_3/3(Z), dcdwbdsl_2/3(Z), dcdwbdsl_1/3(Z)
  Sum7/1 -> dcdpfint/1
  dclpfint1/1 -> Sum7/2
  dclpfint2/1 -> Sum7/1
  dcdwbdsl_2/1(Interp Value) -> dclpfint2/2
  dcdwbdsl_3/1(Interp Value) -> dclpfint2/1, dclpfint1/1
  dcdwbdsl_1/1(Interp Value) -> dclpfint1/2
  dsr/1 -> cd_sp_int/5(dsr), dcdwbdsl_1/1(X), dcdwbdsl_/1(X)
  mach/1 -> dcdwbdsl_/3(Z), dcdwbdsl1/3(Z), dcdwbdsb/3(Z), dcdwbdsl/3(Z)
  dcdwbdsl/1(Interp Value) -> Sum1/2
  alpha/1 -> dcdwbdsl_2/2(Y), dcdwbdsl_1/2(Y), cd_sp_int/2(alpha), dcdwbdsl_3/2(Y), dcdwbdsl_/2(Y), dcdwbdsl/2(Y), dcdwbdsl1/2(Y), dcdwbdsb/2(Y), dcdwbdsb_/2(Y)
  dsl/1 -> dcdwbdsl_2/1(X), cd_sp_int/3(dsl), dcdwbdsl/1(X)
  Sum5/1 -> Sum6/2
  Sum1/1 -> Sum6/1
  dcdwbdsl_/1(Interp Value) -> Sum5/1
  Switch7/1 -> dcdpfint/2
  Sum2/1 -> cd_spoil/1
  flap/1 -> cd_sp_int/1(flap), Switch8/2, Switch7/2, cd_sp_int/Enable
  cd_sp_int/1(cd_sp_int) -> Switch7/1
  zero/1 -> Switch7/3
  dsb/1 -> dcdwbdsb_/1(X), dcdwbdsb/1(X), dcdwbdsl_3/1(X), cd_sp_int/4(dsb), dcdwbdsl1/1(X)
  Sum6/1 -> Sum2/1
  Switch8/1 -> cd_sb/1
  dcdpfint/1 -> Sum2/2, cd_sp_int_df/1

== system gtm_aeromodel/get aero forces and moments/AERODYNAMICS/Force  Coefficients/DRAG /CDTP ==
  mach : Inport  OutDataType=sfix(16)  OutScaling=2^0
  alphat : Inport  Port=2  OutDataType=sfix(16)  OutScaling=2^0
  Product2 : Product  OutDataType=sfix(16)  OutScaling=2^0  SaturateOnIntegerOverflow=on  RndMeth=Zero  InputSameDT=on  OutDataTypeStr=Inherit: Same as first input
  Product3 : Product  OutDataType=sfix(16)  OutScaling=2^0  SaturateOnIntegerOverflow=on  RndMeth=Zero  InputSameDT=on  OutDataTypeStr=Inherit: Same as first input
  Sum1 : Sum  OutDataType=sfix(16)  OutScaling=2^0  SaturateOnIntegerOverflow=on  InputSameDT=on  OutDataTypeStr=Inherit: Same as first input
  Sum2 : Sum  OutDataType=sfix(16)  OutScaling=2^0  SaturateOnIntegerOverflow=on  InputSameDT=on  OutDataTypeStr=Inherit: Same as first input
  cdt1 : Subsystem  mask(1-D Table){z=cdt1x_mach, tab=cdt1}
      mask prompts: z "Z vector:"; tab "Table:"
      mask help: 1-D Table Look Up. Enter monotonic Z vector amd table. See the help for more info.
      mask Help: The Z vector must be monotonic.  Z indexes into the columns of the 1-D tables.   Table does not extrapolate beyound the break vectors
      mask Display: plot(@2)
  cdt2 : Subsystem  mask(1-D Table){z=cdt2x_mach, tab=cdt2}
      mask prompts: z "Z vector:"; tab "Table:"
      mask help: 1-D Table Look Up. Enter monotonic Z vector amd table. See the help for more info.
      mask Help: The Z vector must be monotonic.  Z indexes into the columns of the 1-D tables.   Table does not extrapolate beyound the break vectors
      mask Display: plot(@2)
  cdto : Subsystem  mask(1-D Table){z=cdtox_mach, tab=cdto}
      mask prompts: z "Z vector:"; tab "Table:"
      mask help: 1-D Table Look Up. Enter monotonic Z vector amd table. See the help for more info.
      mask Help: The Z vector must be monotonic.  Z indexes into the columns of the 1-D tables.   Table does not extrapolate beyound the break vectors
      mask Display: plot(@2)
  cdtp : Outport  OutDataType=sfix(16)  OutScaling=2^0  InitialOutput=0
  wires:
  mach/1 -> cdt2/1(Z), cdt1/1(Z), cdto/1(Z)
  Sum1/1 -> Product2/1
  alphat/1 -> Product2/2, Product3/2
  cdt2/1(Interp Value) -> Product3/1
  Product3/1 -> Sum1/2
  cdt1/1(Interp Value) -> Sum1/1
  Product2/1 -> Sum2/2
  Sum2/1 -> cdtp/1
  cdto/1(Interp Value) -> Sum2/1

== system gtm_aeromodel/get aero forces and moments/AERODYNAMICS/Force  Coefficients/DRAG /CDWB ==
  alpha : Inport  OutDataType=sfix(16)  OutScaling=2^0
  mach : Inport  Port=2  OutDataType=sfix(16)  OutScaling=2^0
  flap : Inport  Port=3  OutDataType=sfix(16)  OutScaling=2^0
  flex : Inport  Port=4  OutDataType=sfix(16)  OutScaling=2^0
  altitude : Inport  Port=5  OutDataType=sfix(16)  OutScaling=2^0
  dsb : Inport  Port=6  OutDataType=sfix(16)  OutScaling=2^0
  CDWBFLEX : Subsystem  TreatAsAtomicUnit=on
  Sum1 : Sum  OutDataType=sfix(16)  OutScaling=2^0  SaturateOnIntegerOverflow=on  InputSameDT=on  OutDataTypeStr=Inherit: Same as first input
  Switch5 : Switch  Threshold=0.5  SaturateOnIntegerOverflow=on  InputSameDT=on
  Switch6 : Switch  Threshold=0.5  SaturateOnIntegerOverflow=on  InputSameDT=on
  Switch7 : Switch  Threshold=0.5  SaturateOnIntegerOverflow=on  InputSameDT=on
  cd_flap_ : Subsystem  TreatAsAtomicUnit=on
  cdwb_clean : Subsystem  mask(2-D Table){y=cdwbx_FALPHA, z=cdwby_FMACH, tab=cdwb}
      mask prompts: y "Y vector:"; z "Z vector:"; tab "Table:"
      mask help: 2-D Table Look Up. Enter monotonic Y and Z vectors and a matrix of 2-D tables. See the help for more info.
      mask Help: The Y and Z vectors must be monotonic.  Y  indexes into the columns of the 2-D table & Z indexes into the rows of the 2-D tables.   The input values are y and z respectively (e.g., top port = y).
      mask Display: plot(-10,-10,110,110,[90,50,10],[90,40,30],[90,50,10],[50,26,20],[90,50,10],[22,13,10])
  zero : Constant  Value=0.0  OutDataType=sfix(16)  OutScaling=2^0
  zero1 : Constant  Value=0.0  OutDataType=sfix(16)  OutScaling=2^0
  zero2 : Constant  Value=0.0  OutDataType=sfix(16)  OutScaling=2^0
  cdwb : Outport  OutDataType=sfix(16)  OutScaling=2^0  InitialOutput=0
  cd_flap : Outport  Port=2  OutDataType=sfix(16)  OutScaling=2^0  InitialOutput=0
  dcdsbfint : Outport  Port=3  OutDataType=sfix(16)  OutScaling=2^0  InitialOutput=0
  wires:
  alpha/1 -> cd_flap_/2(alpha), cdwb_clean/1(Y), CDWBFLEX/1(alpha)
  mach/1 -> cdwb_clean/2(Z), CDWBFLEX/2(Mach)
  altitude/1 -> CDWBFLEX/3(altitude)
  cd_flap_/1(cd_flap) -> Switch5/1
  flap/1 -> cd_flap_/1(flap), cd_flap_/Enable, Switch5/2, Switch7/2
  CDWBFLEX/1(dcdflex) -> Switch6/1
  flex/1 -> CDWBFLEX/Enable, Switch6/2
  zero1/1 -> Switch6/3
  Switch6/1 -> Sum1/2
  Sum1/1 -> cdwb/1
  dsb/1 -> cd_flap_/3(dsb)
  Switch5/1 -> cd_flap/1
  cdwb_clean/1(Interp Value) -> Sum1/1
  zero/1 -> Switch5/3
  zero2/1 -> Switch7/3
  cd_flap_/2(dcdsbfint) -> Switch7/1
  Switch7/1 -> dcdsbfint/1

== system gtm_aeromodel/get aero forces and moments/AERODYNAMICS/Force  Coefficients/DRAG /DCDDEL ==
  elev : Inport  OutDataType=sfix(16)  OutScaling=2^0
  alphat : Inport  Port=2  OutDataType=sfix(16)  OutScaling=2^0
  mach : Inport  Port=3  OutDataType=sfix(16)  OutScaling=2^0
  dcdde_ : Subsystem  mask(1-2-3 Table){@1=dcddex_FELE, @2=dcddey_ALPHAT, @3=dcddez_FMACH, @4=dcdde}
      mask prompts: @1 "X vector:"; @2 "Y vector:"; @3 "Z vector:"; @4 "Table:"
      mask help: 3-D Table Look Up. Enter monotonic X, Y and Z vectors and a matrix of 2-D tables. See the help for more info.
      mask init:
      | x=@1;y=@2;z=@3;tab=@4;
      mask Help: The X, Y and Z vectors must be monotonic.   The 3-D table is a horizontal concatenation of  2-D tables.  X  indexes into the columns of the 2-D tables & Y indexes into the rows of the 2-D tables.  Z indexes into the table levels (starting with the 1st 2-D table).   The input values are x, y and z respectively (e.g., top port = x).
      mask Display: plot([0 2 2 0 0],[0 0 2 2 0],[0 2 2.9 0.95 0],[2 2 2.7 2.7 2],[2 2.9 2.9 2 2],[0 0.85 2.7 2 0])
  dcdde : Outport  OutDataType=sfix(16)  OutScaling=2^0  InitialOutput=0
  wires:
  dcdde_/1(Interp Value) -> dcdde/1
  mach/1 -> dcdde_/3(Z)
  elev/1 -> dcdde_/1(X)
  alphat/1 -> dcdde_/2(Y)
